simulink library "Simple_lib"  (R2018b)
settings: Solver=ode45  StartTime=0.0  StopTime=10.0  RelTol=1e-3  EnableMultiTasking=on
undefined symbols (not defined in the file or in its folder): Acceptance, beta, C, C_J, C_P, c_wall, dGain, DiscIntNeverNeededParam, Duplex, Electrical_lib, grab, h_fe, i, i3, K_T, Kman, KmanCE, mu_s, n_rev, R_arm, Simplex, systemTs, tau_0, TinIC, Ts, w_0, wallMass, Watch_lib
libraries: $bdroot x407, PlantUtilityBlockset_lib x30, peGeneralControl x22, simulink x11
(part 5 of 14)

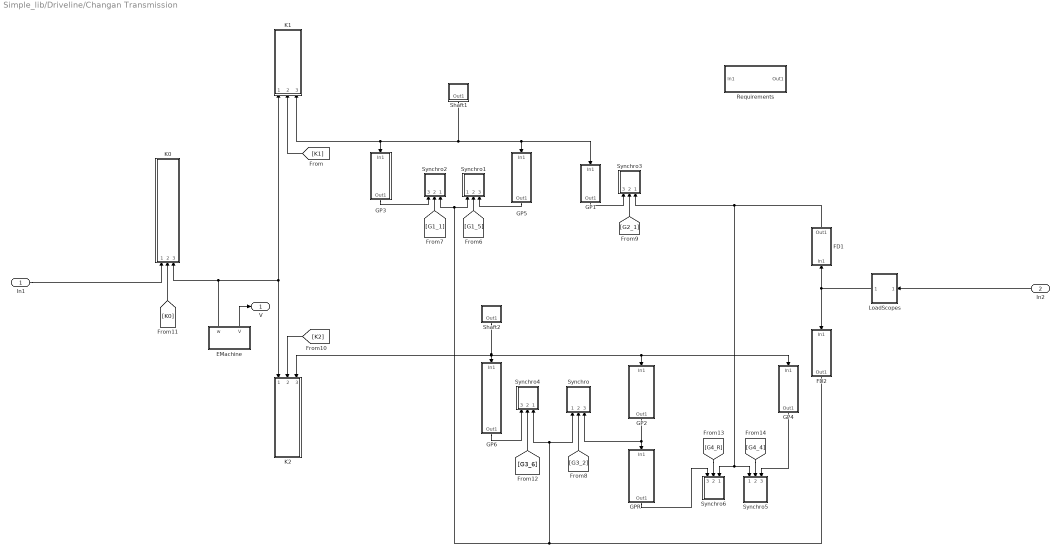
== system Simple_lib/Driveline/Changan Transmission ==
  In1 : Inport
  In2 : Inport  Port=2
  EMachine : Subsystem  AncestorBlock=PlantUtilityBlockset_lib/Electrical/EMachine
  FD1 : Subsystem  AncestorBlock=PlantUtilityBlockset_lib/Driveline/GearPair  mask{n_i=75, n_o=16}
      mask prompts: n_i "Number of input teeth"; n_o "Number of output teeth"
      mask Display:
      | plot([-n_i -5],[0 0]);
      | plot([5 n_o],[0 0]);
      | 
      | patch(-[3 3 5 5],[-1  1 1 -1]*(n_i+n_o));
      | patch([3 3 5 5],[-1  1 1 -1]*(n_i+n_o));
  FD2 : Subsystem  AncestorBlock=PlantUtilityBlockset_lib/Driveline/GearPair  mask{n_i=75, n_o=22}
      mask prompts: n_i "Number of input teeth"; n_o "Number of output teeth"
      mask Display:
      | plot([-n_i -5],[0 0]);
      | plot([5 n_o],[0 0]);
      | 
      | patch(-[3 3 5 5],[-1  1 1 -1]*(n_i+n_o));
      | patch([3 3 5 5],[-1  1 1 -1]*(n_i+n_o));
  GP1 : Subsystem  AncestorBlock=PlantUtilityBlockset_lib/Driveline/GearPair  mask{n_i=17, n_o=59}
      mask prompts: n_i "Number of input teeth"; n_o "Number of output teeth"
      mask Display:
      | plot([-n_i -5],[0 0]);
      | plot([5 n_o],[0 0]);
      | 
      | patch(-[3 3 5 5],[-1  1 1 -1]*(n_i+n_o));
      | patch([3 3 5 5],[-1  1 1 -1]*(n_i+n_o));
  GP2 : Subsystem  AncestorBlock=PlantUtilityBlockset_lib/Driveline/GearPair  mask{n_i=19, n_o=55}
      mask prompts: n_i "Number of input teeth"; n_o "Number of output teeth"
      mask Display:
      | plot([-n_i -5],[0 0]);
      | plot([5 n_o],[0 0]);
      | 
      | patch(-[3 3 5 5],[-1  1 1 -1]*(n_i+n_o));
      | patch([3 3 5 5],[-1  1 1 -1]*(n_i+n_o));
  GP3 : Subsystem  AncestorBlock=PlantUtilityBlockset_lib/Driveline/GearPair  mask{n_i=i3, n_o=49}
      mask prompts: n_i "Number of input teeth"; n_o "Number of output teeth"
      settings: AttributesFormatString=|
      | n_i = %<n_i>
      | n_o = %<n_o>
      mask Display:
      | plot([-n_i -5],[0 0]);
      | plot([5 n_o],[0 0]);
      | 
      | patch(-[3 3 5 5],[-1  1 1 -1]*(n_i+n_o));
      | patch([3 3 5 5],[-1  1 1 -1]*(n_i+n_o));
  "GP4 " : Subsystem  AncestorBlock=PlantUtilityBlockset_lib/Driveline/GearPair  mask{n_i=38, n_o=39}
      mask prompts: n_i "Number of input teeth"; n_o "Number of output teeth"
      mask Display:
      | plot([-n_i -5],[0 0]);
      | plot([5 n_o],[0 0]);
      | 
      | patch(-[3 3 5 5],[-1  1 1 -1]*(n_i+n_o));
      | patch([3 3 5 5],[-1  1 1 -1]*(n_i+n_o));
  GP5 : Subsystem  AncestorBlock=PlantUtilityBlockset_lib/Driveline/GearPair  mask{n_i=38, n_o=43}
      mask prompts: n_i "Number of input teeth"; n_o "Number of output teeth"
      mask Display:
      | plot([-n_i -5],[0 0]);
      | plot([5 n_o],[0 0]);
      | 
      | patch(-[3 3 5 5],[-1  1 1 -1]*(n_i+n_o));
      | patch([3 3 5 5],[-1  1 1 -1]*(n_i+n_o));
  GP6 : Subsystem  AncestorBlock=PlantUtilityBlockset_lib/Driveline/GearPair  mask{n_i=38, n_o=37}
      mask prompts: n_i "Number of input teeth"; n_o "Number of output teeth"
      mask Display:
      | plot([-n_i -5],[0 0]);
      | plot([5 n_o],[0 0]);
      | 
      | patch(-[3 3 5 5],[-1  1 1 -1]*(n_i+n_o));
      | patch([3 3 5 5],[-1  1 1 -1]*(n_i+n_o));
  GPR : Subsystem  AncestorBlock=PlantUtilityBlockset_lib/Driveline/GearPair  mask{n_i=55, n_o=48}
      mask prompts: n_i "Number of input teeth"; n_o "Number of output teeth"
      mask Display:
      | plot([-n_i -5],[0 0]);
      | plot([5 n_o],[0 0]);
      | 
      | patch(-[3 3 5 5],[-1  1 1 -1]*(n_i+n_o));
      | patch([3 3 5 5],[-1  1 1 -1]*(n_i+n_o));
  K0 : Subsystem  AncestorBlock="PlantUtilityBlockset_lib/Driveline/Pseudo Locking  Clutch"
      mask Display:
      | patch([0 1 1 0],[1 1 .9 .9]);
      | patch([0 1 1 0],-[1 1 .9 .9]);
  K1 : Subsystem  AncestorBlock="PlantUtilityBlockset_lib/Driveline/Pseudo Locking  Clutch"
      mask Display:
      | patch([0 1 1 0],[1 1 .9 .9]);
      | patch([0 1 1 0],-[1 1 .9 .9]);
  K2 : Subsystem  AncestorBlock="PlantUtilityBlockset_lib/Driveline/Pseudo Locking  Clutch"
      mask Display:
      | patch([0 1 1 0],[1 1 .9 .9]);
      | patch([0 1 1 0],-[1 1 .9 .9]);
  LoadScopes : Subsystem  AncestorBlock=PlantUtilityBlockset_lib/Utility/Scopes
      mask Display:
      | plot( [-1 1 1 -1 -1], [-1 -1 1 1 -1] );
      | plot( 0.6*[-1 1 1 -1 -1], 0.3 + 0.5*[-1 -1 1 1 -1] );
  Requirements : Subsystem
  Shaft1 : Subsystem  AncestorBlock=PlantUtilityBlockset_lib/Driveline/InertialState
      mask Display:
      | %color('white');
      | %plot([-1 4],[1 1]);
      | %plot([-1 4],[-1 -1]);
      | %color('black')
      | %plot([1 4],[0 0]);
      | plot([-1 -.9 -.5 0 .5 .9 1  .9  .5  0 -.5 -.9 -1],      [ 0  .5 .9 1 .9 .5 0 -.5 -.9 -1 -.9 -.5  0]);
      | %plot([4 4.5 4.5 4],[0 -0.25 0.25 0])
  Shaft2 : Subsystem  AncestorBlock=PlantUtilityBlockset_lib/Driveline/InertialState
      mask Display:
      | %color('white');
      | %plot([-1 4],[1 1]);
      | %plot([-1 4],[-1 -1]);
      | %color('black')
      | %plot([1 4],[0 0]);
      | plot([-1 -.9 -.5 0 .5 .9 1  .9  .5  0 -.5 -.9 -1],      [ 0  .5 .9 1 .9 .5 0 -.5 -.9 -1 -.9 -.5  0]);
      | %plot([4 4.5 4.5 4],[0 -0.25 0.25 0])
  Synchro : Subsystem
      mask Display:
      | %color('black')
      | %patch([-1 0 0 -1], [1 .9 1 .9]);
      | patch([1 1 0.4 -0.4 -1 -1], [1 .6 -.2 -.2 .6 1]);
      | patch([1 1 0.4 -0.4 -1 -1], -[1 0 .8 .8 0 1]);
      | color('white');
      | plot([-1 -1],[-1 1]);
      | plot([1 1],[-1 1]);
  Synchro1 : Subsystem
      mask Display:
      | %color('black')
      | %patch([-1 0 0 -1], [1 .9 1 .9]);
      | patch([1 1 0.4 -0.4 -1 -1], [1 .6 -.2 -.2 .6 1]);
      | patch([1 1 0.4 -0.4 -1 -1], -[1 0 .8 .8 0 1]);
      | color('white');
      | plot([-1 -1],[-1 1]);
      | plot([1 1],[-1 1]);
  Synchro2 : Subsystem
      mask Display:
      | %color('black')
      | %patch([-1 0 0 -1], [1 .9 1 .9]);
      | patch([1 1 0.4 -0.4 -1 -1], [1 .6 -.2 -.2 .6 1]);
      | patch([1 1 0.4 -0.4 -1 -1], -[1 0 .8 .8 0 1]);
      | color('white');
      | plot([-1 -1],[-1 1]);
      | plot([1 1],[-1 1]);
  Synchro3 : Subsystem
      mask Display:
      | %color('black')
      | %patch([-1 0 0 -1], [1 .9 1 .9]);
      | patch([1 1 0.4 -0.4 -1 -1], [1 .6 -.2 -.2 .6 1]);
      | patch([1 1 0.4 -0.4 -1 -1], -[1 0 .8 .8 0 1]);
      | color('white');
      | plot([-1 -1],[-1 1]);
      | plot([1 1],[-1 1]);
  Synchro4 : Subsystem
      mask Display:
      | %color('black')
      | %patch([-1 0 0 -1], [1 .9 1 .9]);
      | patch([1 1 0.4 -0.4 -1 -1], [1 .6 -.2 -.2 .6 1]);
      | patch([1 1 0.4 -0.4 -1 -1], -[1 0 .8 .8 0 1]);
      | color('white');
      | plot([-1 -1],[-1 1]);
      | plot([1 1],[-1 1]);
  Synchro5 : Subsystem
      mask Display:
      | %color('black')
      | %patch([-1 0 0 -1], [1 .9 1 .9]);
      | patch([1 1 0.4 -0.4 -1 -1], [1 .6 -.2 -.2 .6 1]);
      | patch([1 1 0.4 -0.4 -1 -1], -[1 0 .8 .8 0 1]);
      | color('white');
      | plot([-1 -1],[-1 1]);
      | plot([1 1],[-1 1]);
  Synchro6 : Subsystem
      mask Display:
      | %color('black')
      | %patch([-1 0 0 -1], [1 .9 1 .9]);
      | patch([1 1 0.4 -0.4 -1 -1], [1 .6 -.2 -.2 .6 1]);
      | patch([1 1 0.4 -0.4 -1 -1], -[1 0 .8 .8 0 1]);
      | color('white');
      | plot([-1 -1],[-1 1]);
      | plot([1 1],[-1 1]);
  V : Outport
  wires:
  EMachine/2(w) -> K2/1(w_in), K1/1(w_in), K0/3(w_out)
  Shaft1/1(Out1) -> K1/3(w_out), GP3/1(In1), GP1/1(In1), GP5/1(In1)
  GP3/1(Out1) -> Synchro2/3(w_out)
  GP1/1(Out1) -> Synchro3/3(w_out)
  GP2/1(Out1) -> GPR/1(In1), Synchro/3(w_out)
  [K1] -> K1/2(cap)
  [K0] -> K0/2(cap)
  [K2] -> K2/2(cap)
  [G2_1] -> Synchro3/2(cap)
  [G3_2] -> Synchro/2(cap)
  [G1_1] -> Synchro2/2(cap)
  [G1_5] -> Synchro1/2(cap)
  GP5/1(Out1) -> Synchro1/3(w_out)
  FD1/1(Out1) -> Synchro6/1(w_in), Synchro5/1(w_in), Synchro3/1(w_in)
  GP6/1(Out1) -> Synchro4/3(w_out)
  [G3_6] -> Synchro4/2(cap)
  Shaft2/1(Out1) -> K2/3(w_out), "GP4 "/1(In1), GP2/1(In1), GP6/1(In1)
  "GP4 "/1(Out1) -> Synchro5/3(w_out)
  [G4_4] -> Synchro5/2(cap)
  [G4_R] -> Synchro6/2(cap)
  GPR/1(Out1) -> Synchro6/3(w_out)
  EMachine/1(V) -> V/1
  FD2/1(Out1) -> Synchro1/1(w_in), Synchro2/1(w_in), Synchro4/1(w_in), Synchro/1(w_in)
  LoadScopes/1(Out1) -> FD1/1(In1), FD2/1(In1)
  In2/1 -> LoadScopes/1(In1)
  In1/1 -> K0/1(w_in)

== system Simple_lib/Driveline/Clutch ==
  note: {\bfSimple Clutch}
      | Clutch torque is a sigmoidal function of speed difference.
  K : Inport
  in : Inport  Port=2
  T : Inport  Port=3
  Friction : $bdroot/Rotational/Friction  grab=.03  s=.2  Ki=1
  Saturation : Saturate  UpperLimit=inf  LowerLimit=0
      settings: AttributesFormatString=|
      | %<UpperLimit>
      | %<LowerLimit>
  Terminator : Terminator
  from : $bdroot/Rotational/Lump  w_0=w_0  max_accel=inf  conserved_quantity_name=Momentum  energy_name=Energy
  out : Outport
  wires:
  K/1 -> Saturation/1
  in/1 -> Friction/1
  T/1 -> Terminator/1
  Saturation/1 -> Friction/2
  from/1 -> out/1, Friction/3

== system Simple_lib/Driveline/Compliant Wheel_wv ==
  w : Inport
  r : Inport  Port=2
  Bus Creator : BusCreator  Inputs=2
  Bus Selector : BusSelector  OutputSignals=F,M
  Times : Product  Inputs=**
  Times1 : Product  Inputs=**
  Times2 : Product  Inputs=**
  _out : $bdroot/Translational/_out  Tag=Electrical  Level=v  Flow=F
  in : $bdroot/Rotational/_in  Level=w  Flow=Tq
  v : Outport
  wires:
  Bus Selector/1 -> Times1/2  "<F>"
  Bus Selector/2 -> Times2/2  "<M>"
  in/1 -> Times/1
  Times/1 -> _out/1
  _out/2 -> Bus Selector/1
  Bus Creator/1 -> in/2
  w/1 -> in/1
  _out/1 -> v/1
  r/1 -> Times/2, Times1/1, Times2/1
  Times1/1 -> Bus Creator/1  "tau"
  Times2/1 -> Bus Creator/2  "J"

== system Simple_lib/Driveline/Differential ==
  In1 : Inport
  BiGain : $bdroot/Rotational/BiGain  k_level=-1  k_flow=-1
      settings: AttributesFormatString="%<k_flow>   %<k_pot>"
  First : $bdroot/Driveline/GearPair  n_i=r*100  n_o=100
  InertialState : $bdroot/Rotational/Lump  w_0=0  max_accel=inf
  Sum : Sum  Inputs=|++
  Sum1 : Sum  Inputs=|++
  Out1 : Outport
  Out2 : Outport  Port=2
  wires:
  BiGain/1 -> Sum/2
  Sum1/1 -> Out2/1
  Sum/1 -> Out1/1
  InertialState/1 -> BiGain/1, Sum1/2
  First/1 -> Sum1/1, Sum/1
  In1/1 -> First/1

== system Simple_lib/Driveline/Drag ==
  In1 : Inport
  A : Gain  Gain=2
  Bus Creator : BusCreator  Inputs=2
  Bus Selector : BusSelector  OutputSignals=i
  Cd : Gain  Gain=0.3
  Gain2 : Gain  Gain=-1/2
  Ground : Ground
  Multiply : Product  Inputs=3
  Sign : Signum
  _at : $bdroot/Translational/_in  Level=v  Flow=F
  rho : Gain
  wires:
  In1/1 -> Bus Selector/1
  _at/1 -> Multiply/2, Multiply/3, Sign/1
  Sign/1 -> Multiply/1
  Multiply/1 -> Gain2/1
  Cd/1 -> A/1
  A/1 -> rho/1
  Gain2/1 -> Cd/1
  rho/1 -> Bus Creator/1  "F"
  Bus Selector/1 -> _at/1  "<i>"
  Bus Creator/1 -> _at/2
  Ground/1 -> Bus Creator/2  "M"

== system Simple_lib/Driveline/EndStop ==
  In1 : Inport
  In2 : Inport  Port=2
  1/R1 : Gain  Gain=-1
  1/R2 : Gain  Gain=-1
  1/R3 : Gain  Gain=k
  1/R4 : Gain  Gain=k
  Compare To Zero : simulink/Logic and Bit Operations/Compare To Zero  relop=~=  OutDataTypeStr=boolean
  Dead Zone : DeadZone  LowerValue=-0.01  UpperValue=0.31  SaturateOnIntegerOverflow=on
  Discrete-Time Integrator1 : DiscreteIntegrator  gainval=1  SampleTime=Ts  ICPrevOutput=DiscIntNeverNeededParam  ICPrevScaledInput=DiscIntNeverNeededParam
  Input : $bdroot/Utility/Input  Level=V  Flow=I
  Input1 : $bdroot/Utility/Input  Level=V  Flow=I
  Multiply : Product
  Sum : Sum  Inputs=+|+
  Sum1 : Sum  Inputs=|++
  wires:
  Compare To Zero/1 -> Multiply/1
  Multiply/1 -> 1/R4/1
  1/R4/1 -> Sum1/2
  1/R3/1 -> Sum1/1
  1/R1/1 -> Input1/2
  Input1/1 -> Sum/2
  In2/1 -> Input1/1
  Sum/1 -> Discrete-Time Integrator1/1, Multiply/2
  1/R2/1 -> Sum/1
  Input/1 -> 1/R2/1
  In1/1 -> Input/1
  Discrete-Time Integrator1/1 -> Dead Zone/1
  Dead Zone/1 -> 1/R3/1, Compare To Zero/1
  Sum1/1 -> 1/R1/1, Input/2

== system Simple_lib/Driveline/Engine ==
  Ped : Inport
  Crank : $bdroot/Driveline/MeanTorqueMapModel  SystemSampleTime=-1
  Flywheel : $bdroot/Rotational/Lump  w_0=w_0  max_accel=inf  conserved_quantity_name=Momentum  energy_name=Energy
  Inertia : $bdroot/Rotational/Inertia  I=0.1
      settings: AttributesFormatString=%<I> kgm^2
  M : $bdroot/Rotational/M1  SystemSampleTime=-1
  w : Outport
  wires:
  Flywheel/1 -> Inertia/1, M/1, Crank/2
  M/1 -> w/1
  Ped/1 -> Crank/1

== system Simple_lib/Driveline/FailingClutch ==
  note: {\bfClutch}
      | Passes the smaller of the input torque and its (non-negative) capacity K (Kappa).
  K : Inport
  in : Inport  Port=2
  T : Inport  Port=3
  Abs1 : Abs
  Complex to Real-Imag1 : ComplexToRealImag
  Discrete-Time Integrator : DiscreteIntegrator  gainval=1  InitialCondition=w_0  SampleTime=-1  LowerSaturationLimit=0  ICPrevOutput=DiscIntNeverNeededParam  ICPrevScaledInput=DiscIntNeverNeededParam
  Filtered Derivative (Discrete or Continuous) : peGeneralControl/Filtered Derivative (Discrete or Continuous)  K=1  T=Ts*20  B=inf  A=-inf  minRatio=10  Ts=-1
  Gain : Gain  Gain=-1
  Gain1 : Gain  Gain=+1
  Ground : Ground
  MinMax1 : MinMax  Inputs=2
  Multiply : Product  Inputs=*/
  Product1 : Product
  Product2 : Product
  Real-Imag to Complex1 : RealImagToComplex
  Saturation1 : Saturate  UpperLimit=inf  LowerLimit=0
      settings: AttributesFormatString=|
      | %<UpperLimit>
      | %<LowerLimit>
  Sign1 : Signum
  Sum1 : Sum  Inputs=|-+
  Terminator : Terminator
  _in : $bdroot/Utility/Input  Level=w  Flow=Tq
  _out : $bdroot/Utility/Output  Tag=Electrical  Level=w  Flow=Tq
  out : Outport
  wires:
  Gain/1 -> Discrete-Time Integrator/1  "dw_on"
  Filtered Derivative (Discrete or Continuous)/1 -> Gain1/1
  Product2/1 -> Sum1/1  "Tq_I"
  Gain1/1 -> Product2/1  "dw_in"
  Complex to Real-Imag1/2 -> Product2/2, Multiply/2  "Inertia"
  Multiply/1 -> Gain/1
  Ground/1 -> Real-Imag to Complex1/2
  Sum1/1 -> Sign1/1, Abs1/1  "Tq_needed"
  Saturation1/1 -> MinMax1/1
  Sign1/1 -> Product1/2
  Abs1/1 -> MinMax1/2
  K/1 -> Saturation1/1
  MinMax1/1 -> Product1/1
  _out/2 -> Complex to Real-Imag1/1
  Real-Imag to Complex1/1 -> _in/2
  _out/1 -> out/1
  _in/1 -> Filtered Derivative (Discrete or Continuous)/1  "w_in"
  Discrete-Time Integrator/1 -> _out/1  "w_out"
  Product1/1 -> Multiply/1, Real-Imag to Complex1/1  "Tq_trn"
  in/1 -> _in/1
  T/1 -> Terminator/1
  Complex to Real-Imag1/1 -> Sum1/2  "Tq_Re"

== system Simple_lib/Driveline/GearPair ==
  In1 : Inport
  Bus Creator : BusCreator  Inputs=2
  Bus Selector : BusSelector  OutputSignals=tau,J
  _in : $bdroot/Rotational/_in  Level=w  Flow=tau
  _out : $bdroot/Rotational/_out  Tag=Electrical  Level=w  Flow=tau
  ratio : Gain  Gain=n_i/n_o
  ratio1 : Gain  Gain=n_i/n_o
  ratio2 : Gain  Gain=n_i/n_o
  speed ratio : Gain  Gain=n_i/n_o
  Out1 : Outport
  wires:
  _in/1 -> speed ratio/1
  speed ratio/1 -> _out/1
  Bus Creator/1 -> _in/2
  In1/1 -> _in/1
  _out/1 -> Out1/1
  _out/2 -> Bus Selector/1
  Bus Selector/1 -> ratio/1  "<tau>"
  ratio/1 -> Bus Creator/1  "tau"
  Bus Selector/2 -> ratio2/1  "<J>"
  ratio2/1 -> ratio1/1
  ratio1/1 -> Bus Creator/2  "J"

== system Simple_lib/Driveline/GearPair  ==
  In1 : Inport
  Pull : PlantUtilityBlockset_lib/Utility/Pull  Tag=Electrical  SystemSampleTime=-1
  Push : PlantUtilityBlockset_lib/Utility/Push  SystemSampleTime=-1
  ratio : Gain  Gain=n_i/n_o
  speed ratio : Gain  Gain=n_i/n_o
  Out1 : Outport
  wires:
  Pull/1 -> Out1/1
  In1/1 -> Push/1
  ratio/1 -> Push/2
  Pull/2 -> ratio/1
  speed ratio/1 -> Pull/1
  Push/1 -> speed ratio/1

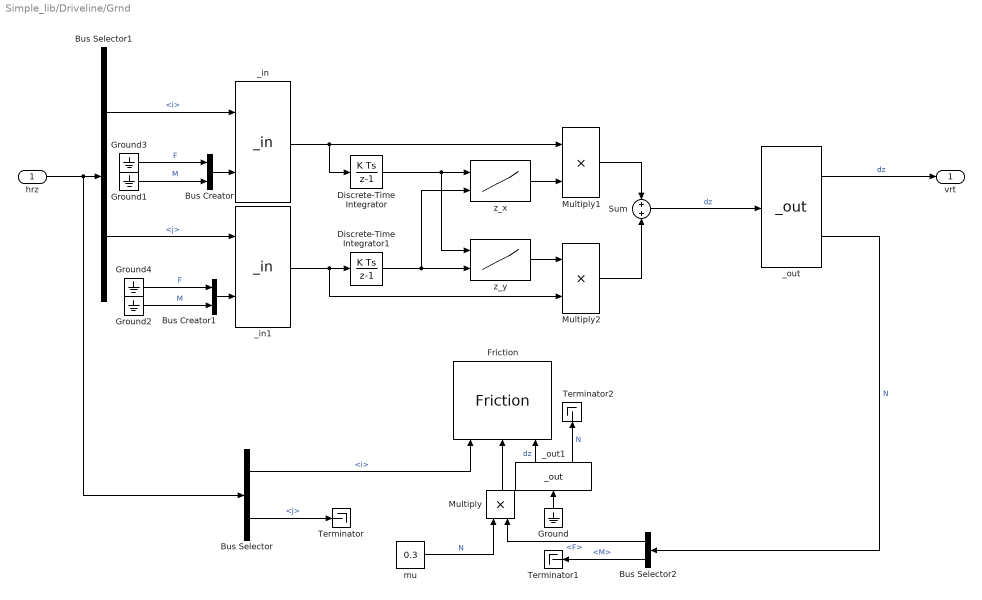
== system Simple_lib/Driveline/Grnd ==
  hrz : Inport
  Bus Creator : BusCreator  Inputs=2
  Bus Creator1 : BusCreator  Inputs=2
  Bus Selector : BusSelector  OutputSignals=i,j
  Bus Selector1 : BusSelector  OutputSignals=i,j
  Bus Selector2 : BusSelector  OutputSignals=F,M
  Discrete-Time Integrator : DiscreteIntegrator  SampleTime=-1  ICPrevOutput=DiscIntNeverNeededParam  ICPrevScaledInput=DiscIntNeverNeededParam
  Discrete-Time Integrator1 : DiscreteIntegrator  SampleTime=-1  ICPrevOutput=DiscIntNeverNeededParam  ICPrevScaledInput=DiscIntNeverNeededParam
  Friction : $bdroot/Translational/Friction  grab=0.1  s=1  Ki=0
  Ground{,1..4} (5 alike) : Ground
  Multiply : Product
  Multiply1 : Product
  Multiply2 : Product
  Sum : Sum  Inputs=+|+
  Terminator : Terminator
  Terminator1 : Terminator
  Terminator2 : Terminator
  _in : $bdroot/Translational/_in  Level=v  Flow=F
  _in1 : $bdroot/Translational/_in  Level=v  Flow=F
  _out : $bdroot/Translational/_out  Tag=Electrical  Level=v  Flow=F
  _out1 : $bdroot/Translational/_out  Tag=Electrical  Level=v  Flow=F
  mu : Constant  Value=0.3
  z_x : Lookup_n-D  BreakpointsForDimension1=[1:3]  BreakpointsForDimension2=[1:3]  Table=[4 5 6;16 19 20;10 18 23]*0  InternalRulePriority=Speed  RndMeth=Simplest  InputSameDT=on
  z_y : Lookup_n-D  BreakpointsForDimension1=[1:3]  BreakpointsForDimension2=[1:3]  Table=[4 5 6;16 19 20;10 18 23]*0  InternalRulePriority=Speed  RndMeth=Simplest  InputSameDT=on
  vrt : Outport
  wires:
  Sum/1 -> _out/1  "dz"
  Multiply2/1 -> Sum/2
  Multiply1/1 -> Sum/1
  z_y/1 -> Multiply2/1
  z_x/1 -> Multiply1/2
  Discrete-Time Integrator1/1 -> z_y/2, z_x/2
  Discrete-Time Integrator/1 -> z_x/1, z_y/1
  _in1/1 -> Multiply2/2, Discrete-Time Integrator1/1
  _in/1 -> Discrete-Time Integrator/1, Multiply1/1
  Ground1/1 -> Bus Creator/2  "M"
  Ground/1 -> _out1/1
  Bus Selector/1 -> Friction/1  "<i>"
  hrz/1 -> Bus Selector/1, Bus Selector1/1
  mu/1 -> Multiply/1  "N"
  _out/1 -> vrt/1  "dz"
  _out/2 -> Bus Selector2/1  "N"
  Multiply/1 -> Friction/2
  Bus Selector/2 -> Terminator/1  "<j>"
  Bus Selector2/1 -> Multiply/2  "<F>"
  Bus Selector2/2 -> Terminator1/1  "<M>"
  Bus Selector1/1 -> _in/1  "<i>"
  Bus Selector1/2 -> _in1/1  "<j>"
  _out1/1 -> Friction/3  "dz"
  _out1/2 -> Terminator2/1  "N"
  Bus Creator/1 -> _in/2
  Ground3/1 -> Bus Creator/1  "F"
  Bus Creator1/1 -> _in1/2
  Ground4/1 -> Bus Creator1/1  "F"
  Ground2/1 -> Bus Creator1/2  "M"

== system Simple_lib/Driveline/Hub ==
  in : Inport
  Brake : $bdroot/Driveline/Brake  SystemSampleTime=-1
  Bus Creator : BusCreator  Inputs=2
  Bus Creator1 : BusCreator  Inputs=3
  Bus Selector : BusSelector  OutputSignals=str,brk,rtn,trn
  Bus Selector1 : BusSelector  OutputSignals=i,j,k
  Ground : Ground
  I : $bdroot/Rotational/Inertia  I=1
  Inertia : $bdroot/Translational/Sink  m=0.01
  Terminator2 : Terminator
  out : Outport
  wires:
  Bus Creator1/1 -> Bus Creator/2  "trn"
  Bus Selector1/3 -> Inertia/1, Bus Creator1/3  "<k>"
  Bus Selector1/2 -> Bus Creator1/2  "<j>"
  Bus Selector1/1 -> Bus Creator1/1  "<i>"
  Bus Selector/4 -> Bus Selector1/1  "<trn>"
  Bus Creator/1 -> out/1  "hub"
  in/1 -> Bus Selector/1
  Bus Selector/2 -> Brake/1  "<brk>"
  Ground/1 -> Brake/3
  Bus Selector/3 -> Brake/2, I/1, Bus Creator/1  "<rtn>"
  Bus Selector/1 -> Terminator2/1  "<str>"

== system Simple_lib/Driveline/Inverter_F ==
  note: NB currently 100% efficient!
  Vdc : Inport
  P_req : Inport  Port=2
  Vac : Inport  Port=3
  DivideSafely_1 : Subsystem
  DivideSafely_2 : Subsystem
  Preq_F : Scope
  Simplex : Subsystem  Tag=Electrical  AncestorBlock=PlantUtilityBlockset_lib/Utility/Push  InitFcn=initSimplex
      mask Display:
      | color('white')
      | plot([0 3], [2 2])
      | plot([0 3], [-2 -2])
      | color('black')
      | 
      | plot([0 2 2 3], [1 1 0 0])
      | plot([1 3 2 1 0 2], [0.6 0.6 0.4 0.6 0.4 0.4])
      | patch([1 3 2],[0.6 0.6 0.4],[0,0,0])
      | plot([0 1 1], [1 1 0.6])
      | plot([1 1 0], [0.4 -1 -1])
  Simplex1 : Subsystem  Tag=Electrical  AncestorBlock=PlantUtilityBlockset_lib/Utility/Push  InitFcn=initSimplex
      mask Display:
      | color('white')
      | plot([0 3], [2 2])
      | plot([0 3], [-2 -2])
      | color('black')
      | 
      | plot([0 2 2 3], [1 1 0 0])
      | plot([1 3 2 1 0 2], [0.6 0.6 0.4 0.6 0.4 0.4])
      | patch([1 3 2],[0.6 0.6 0.4],[0,0,0])
      | plot([0 1 1], [1 1 0.6])
      | plot([1 1 0], [0.4 -1 -1])
  wires:
  Vac/1 -> Simplex/1(InPot)
  Vdc/1 -> Simplex1/1(InPot)
  Simplex1/1(OutPot) -> DivideSafely_1/1(den)
  Simplex/1(OutPot) -> DivideSafely_2/2(den)
  DivideSafely_1/1(rat) -> Simplex1/2(InFlow)
  DivideSafely_2/1(rat) -> Simplex/2(InFlow)
  P_req/1 -> Preq_F/1, DivideSafely_1/2(num), DivideSafely_2/1(num)

== system Simple_lib/Driveline/Inverter_R ==
  note: NB currently 100% efficient!
  note: NB currently 100% efficient!
  Vdc : Inport
  P_req : Inport  Port=2
  Vac : Inport  Port=3
  DivideSafely_1 : Subsystem
  DivideSafely_2 : Subsystem
  Preq_R : Scope
  Simplex : Subsystem  Tag=Electrical  AncestorBlock=PlantUtilityBlockset_lib/Utility/Push  InitFcn=initSimplex
      mask Display:
      | color('white')
      | plot([0 3], [2 2])
      | plot([0 3], [-2 -2])
      | color('black')
      | 
      | plot([0 2 2 3], [1 1 0 0])
      | plot([1 3 2 1 0 2], [0.6 0.6 0.4 0.6 0.4 0.4])
      | patch([1 3 2],[0.6 0.6 0.4],[0,0,0])
      | plot([0 1 1], [1 1 0.6])
      | plot([1 1 0], [0.4 -1 -1])
  Simplex1 : Subsystem  Tag=Electrical  AncestorBlock=PlantUtilityBlockset_lib/Utility/Push  InitFcn=initSimplex
      mask Display:
      | color('white')
      | plot([0 3], [2 2])
      | plot([0 3], [-2 -2])
      | color('black')
      | 
      | plot([0 2 2 3], [1 1 0 0])
      | plot([1 3 2 1 0 2], [0.6 0.6 0.4 0.6 0.4 0.4])
      | patch([1 3 2],[0.6 0.6 0.4],[0,0,0])
      | plot([0 1 1], [1 1 0.6])
      | plot([1 1 0], [0.4 -1 -1])
  Test : Scope
  wires:
  Vac/1 -> Simplex/1(InPot)
  Vdc/1 -> Simplex1/1(InPot)
  Simplex1/1(OutPot) -> DivideSafely_1/1(den)
  Simplex/1(OutPot) -> DivideSafely_2/2(den)
  DivideSafely_1/1(rat) -> Test/1, Simplex1/2(InFlow)
  DivideSafely_2/1(rat) -> Simplex/2(InFlow)
  P_req/1 -> Preq_R/1, DivideSafely_1/2(num), DivideSafely_2/1(num)

== system Simple_lib/Driveline/KellyClutch ==
  note: {\bfSeries Clutch}
      | Passes the smaller of the input torque and its capacity.
  K : Inport
  w_in : Inport  Port=2
  T : Inport  Port=3
  Abs : Abs
  Bus Selector : BusSelector  OutputSignals=tau,J
  Discrete-Time Integrator : DiscreteIntegrator  gainval=k_clutch  InitialCondition=max(w_drop,0)  SampleTime=Ts  LimitOutput=on  LowerSaturationLimit=0  ICPrevOutput=DiscIntNeverNeededParam  ICPrevScaledInput=DiscIntNeverNeededParam
  Divide : Product  Inputs=*/
  MinMax : MinMax  Inputs=2
  Product : Product
  Real-Imag to Complex : RealImagToComplex
  Saturation : Saturate  UpperLimit=inf  LowerLimit=0
      settings: AttributesFormatString=|
      | %<UpperLimit>
      | %<LowerLimit>
  Sign : Signum
  Sum : Sum  Inputs=|+-
  Sum1 : Sum  Inputs=|-+
  Terminator : Terminator
  _in : $bdroot/Rotational/_in  Level=w  Flow=tau
  _out : $bdroot/Rotational/_out  Tag=Electrical  Level=w  Flow=tau
  w_out : Outport
  wires:
  ? -> Real-Imag to Complex/2
  Real-Imag to Complex/1 -> _in/2
  _out/1 -> w_out/1
  _in/1 -> Sum/1
  Sum/1 -> _out/1
  MinMax/1 -> Product/2
  K/1 -> Saturation/1
  Abs/1 -> MinMax/1
  Product/1 -> Real-Imag to Complex/1
  Sign/1 -> Product/1
  Sum1/1 -> Divide/1
  Discrete-Time Integrator/1 -> Sum/2
  w_in/1 -> _in/1
  Saturation/1 -> Sum1/1, MinMax/2
  T/1 -> Terminator/1
  _out/2 -> Bus Selector/1, Abs/1, Sign/1
  Bus Selector/1 -> Sum1/2  "<tau>"
  Divide/1 -> Discrete-Time Integrator/1
  Bus Selector/2 -> Divide/2  "<J>"

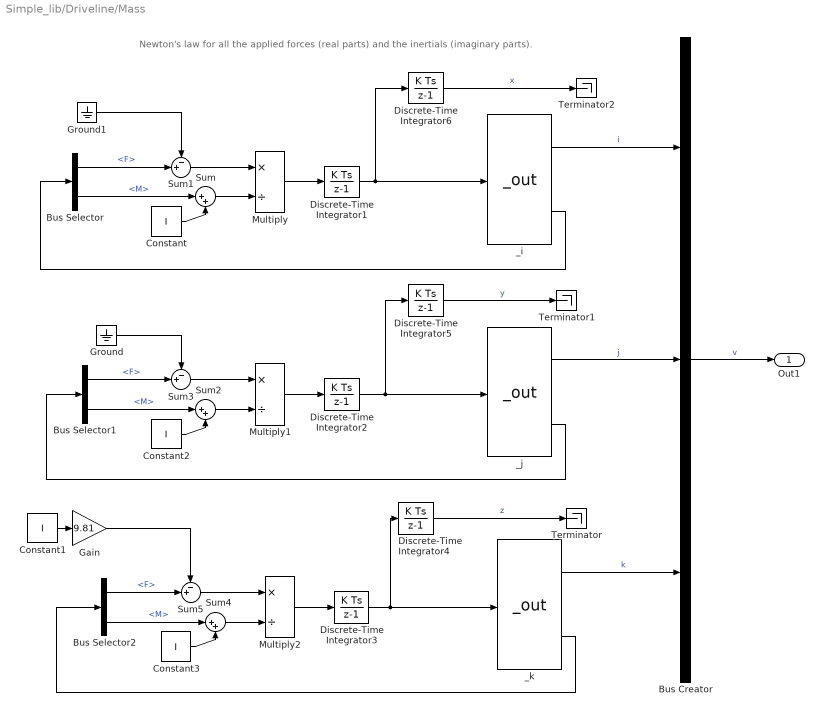
== system Simple_lib/Driveline/Mass ==
  note: Newton's law for all the applied forces (real parts) and the inertials (imaginary parts).
  Bus Creator : BusCreator  Inputs=3
  Bus Selector : BusSelector  OutputSignals=F,M
  Bus Selector1 : BusSelector  OutputSignals=F,M
  Bus Selector2 : BusSelector  OutputSignals=F,M
  Constant{,1..3} (4 alike) : Constant  Value=I
  Discrete-Time Integrator1 : DiscreteIntegrator  gainval=1  InitialCondition=v_0(1)  SampleTime=-1  ICPrevOutput=DiscIntNeverNeededParam  ICPrevScaledInput=DiscIntNeverNeededParam
  Discrete-Time Integrator2 : DiscreteIntegrator  gainval=1  InitialCondition=v_0(2)  SampleTime=-1  ICPrevOutput=DiscIntNeverNeededParam  ICPrevScaledInput=DiscIntNeverNeededParam
  Discrete-Time Integrator{3..6} (4 alike) : DiscreteIntegrator  gainval=1  InitialCondition=v_0(3)  SampleTime=-1  ICPrevOutput=DiscIntNeverNeededParam  ICPrevScaledInput=DiscIntNeverNeededParam
  Gain : Gain  Gain=9.81
  Ground : Ground
  Ground1 : Ground
  Multiply : Product  Inputs=*/
  Multiply1 : Product  Inputs=*/
  Multiply2 : Product  Inputs=*/
  Sum : Sum  Inputs=|++
  Sum1 : Sum  Inputs=-+|
  Sum2 : Sum  Inputs=|++
  Sum3 : Sum  Inputs=-+|
  Sum4 : Sum  Inputs=|++
  Sum5 : Sum  Inputs=-+|
  Terminator : Terminator
  Terminator1 : Terminator
  Terminator2 : Terminator
  _i : $bdroot/Translational/_out  Tag=Electrical  Level=v  Flow=F
  _j : $bdroot/Translational/_out  Tag=Electrical  Level=v  Flow=F
  _k : $bdroot/Translational/_out  Tag=Electrical  Level=v  Flow=F
  Out1 : Outport
  wires:
  Discrete-Time Integrator6/1 -> Terminator2/1  "x"
  Discrete-Time Integrator5/1 -> Terminator1/1  "y"
  Discrete-Time Integrator4/1 -> Terminator/1  "z"
  Ground1/1 -> Sum1/1
  Constant1/1 -> Gain/1
  Gain/1 -> Sum5/1
  Ground/1 -> Sum3/1
  Bus Selector2/2 -> Sum4/1  "<M>"
  Sum5/1 -> Multiply2/1
  Sum4/1 -> Multiply2/2
  Constant3/1 -> Sum4/2
  _k/2 -> Bus Selector2/1
  Bus Selector2/1 -> Sum5/2  "<F>"
  Discrete-Time Integrator3/1 -> _k/1, Discrete-Time Integrator4/1
  Multiply2/1 -> Discrete-Time Integrator3/1
  Bus Selector1/2 -> Sum2/1  "<M>"
  Sum3/1 -> Multiply1/1
  Sum2/1 -> Multiply1/2
  Constant2/1 -> Sum2/2
  _j/2 -> Bus Selector1/1
  Bus Selector1/1 -> Sum3/2  "<F>"
  Discrete-Time Integrator2/1 -> _j/1, Discrete-Time Integrator5/1
  Multiply1/1 -> Discrete-Time Integrator2/1
  _i/1 -> Bus Creator/1  "i"
  _j/1 -> Bus Creator/2  "j"
  Bus Creator/1 -> Out1/1  "v"
  _k/1 -> Bus Creator/3  "k"
  Multiply/1 -> Discrete-Time Integrator1/1
  Discrete-Time Integrator1/1 -> _i/1, Discrete-Time Integrator6/1
  Constant/1 -> Sum/2
  Bus Selector/1 -> Sum1/2  "<F>"
  _i/2 -> Bus Selector/1
  Sum/1 -> Multiply/2
  Sum1/1 -> Multiply/1
  Bus Selector/2 -> Sum/1  "<M>"

== system Simple_lib/Driveline/MeanTorqueMapModel ==
  Ped : Inport
  w : Inport  Port=2
  Bus Creator : BusCreator  Inputs=3
  Gain : Gain  Gain=-1
  Ground : Ground
  Ground1 : Ground
  MeanTorqueMap : Lookup2D  RowIndex=[0,20,30,40,50,60,70,80,90,100]  ColumnIndex=[800,1200,1600,2000,2400,2800,3200,3600,4000,4400,4800]  Table=reshape([-40,215,230,250,245,267,267,267,267,267,-44,117,208,260,279,290,297,301,301,301,-49,85,178,241,282,293,305,308,312,312,-53,66,148,219,275,297,305,312,319,319,-57,44,122,193,260,290,305,319,327,327,-62,29,104,167,238,275,301,323,327,334,-64,10,85,152,223,260,293,319,327,334,-70,-2,66,133,208,256,282,316,327,334,-75,-13,48,119,189,234,267,297,312,319,-79,-22,33,96,171,212,249,279,293,305,-82,-32,18,85,152,193,226,253,267,275],10,11)
  SItoRPM : Gain  Gain=2*pi/60
  _at : $bdroot/Rotational/_in  Level=w  Flow=Tq
  wires:
  Gain/1 -> Bus Creator/1  "tau"
  Ground1/1 -> Bus Creator/2  "c"
  _at/1 -> SItoRPM/1  "w"
  MeanTorqueMap/1 -> Gain/1  "tau_out"
  SItoRPM/1 -> MeanTorqueMap/2  "w_rpm"
  Ground/1 -> Bus Creator/3  "J"
  w/1 -> _at/1  "w"
  Bus Creator/1 -> _at/2
  Ped/1 -> MeanTorqueMap/1

== system Simple_lib/Driveline/Pseudo Locking Clutch ==
  w_in : Inport
  cap : Inport  Port=2
  w_out : Inport  Port=3
  1/R1 : Gain  Gain=-1
  1/R4 : Gain  Gain=-1
  Delay : Delay  DelayLength=1  InitialCondition=0
  Dw : Scope
  Dynamic Friction : Subsystem
  Push_in : Subsystem  AncestorBlock=PlantUtilityBlockset_lib/Utility/Push  InitFcn=initSimplex
      mask Display:
      | color('white')
      | plot([0 3], [2 2])
      | plot([0 3], [-2 -2])
      | color('black')
      | 
      | plot([0 2 2 3], [1 1 0 0])
      | plot([1 3 2 1 0 2], [0.6 0.6 0.4 0.6 0.4 0.4])
      | patch([1 3 2],[0.6 0.6 0.4],[0,0,0])
      | plot([0 1 1], [1 1 0.6])
      | plot([1 1 0], [0.4 -1 -1])
  Push_out : Subsystem  AncestorBlock=PlantUtilityBlockset_lib/Utility/Push  InitFcn=initSimplex
      mask Display:
      | color('white')
      | plot([0 3], [2 2])
      | plot([0 3], [-2 -2])
      | color('black')
      | 
      | plot([0 2 2 3], [1 1 0 0])
      | plot([1 3 2 1 0 2], [0.6 0.6 0.4 0.6 0.4 0.4])
      | patch([1 3 2],[0.6 0.6 0.4],[0,0,0])
      | plot([0 1 1], [1 1 0.6])
      | plot([1 1 0], [0.4 -1 -1])
  Static Friction : Subsystem
  Sum : Sum  Inputs=+|+
  Sum1 : Sum  Inputs=+|+
  Tq_Dyn : Scope
  Tq_stat : Scope
  Tq_trans : Scope
  capacity : Scope
  wires:
  1/R1/1 -> Push_out/2(InFlow)
  cap/1 -> Static Friction/1(cap), Dynamic Friction/2(cap), capacity/1
  Delay/1 -> Static Friction/4(Tq), Tq_trans/1
  Static Friction/1(Tq_stat) -> Sum1/2, Tq_stat/1
  Dynamic Friction/1(Tq_dyn) -> Sum1/1, Tq_Dyn/1
  Push_in/1(OutPot) -> 1/R4/1
  Push_out/1(OutPot) -> Sum/2, Static Friction/3(w)
  Sum/1 -> Static Friction/2(Dw), Dw/1, Dynamic Friction/1(Dw)
  Sum1/1 -> Push_in/2(InFlow), Delay/1, 1/R1/1
  1/R4/1 -> Sum/1
  w_in/1 -> Push_in/1(InPot)
  w_out/1 -> Push_out/1(InPot)

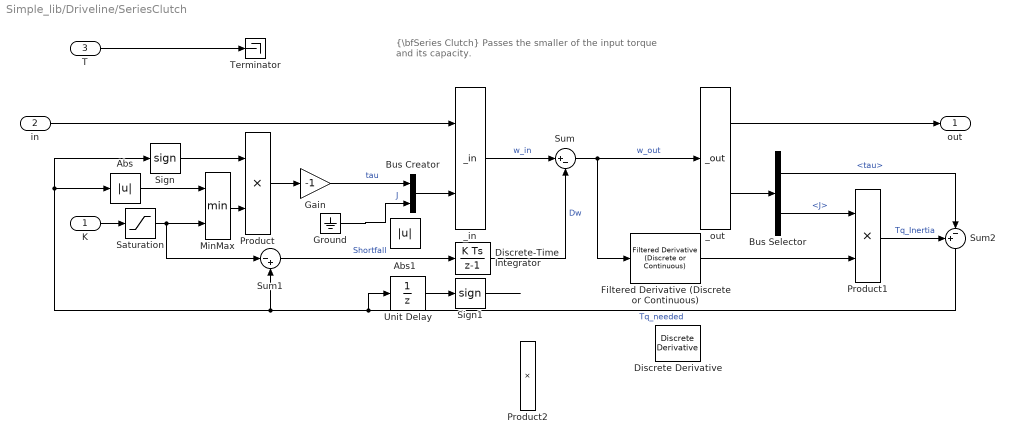
== system Simple_lib/Driveline/SeriesClutch ==
  note: {\bfSeries Clutch}
      | Passes the smaller of the input torque and its capacity.
  K : Inport
  in : Inport  Port=2
  T : Inport  Port=3
  Abs : Abs
  Abs1 : Abs
  Bus Creator : BusCreator  Inputs=2
  Bus Selector : BusSelector  OutputSignals=tau,J
  Discrete Derivative : simulink/Discrete/Discrete Derivative  gainval=1.0  ICPrevScaledInput=0.0  OutMin=[]  OutMax=[]  OutDataType=fixdt(1, 16)  OutScaling=2^-10  DoSatur=off
  Discrete-Time Integrator : DiscreteIntegrator  gainval=20  SampleTime=Ts  LimitOutput=on  LowerSaturationLimit=0  ICPrevOutput=DiscIntNeverNeededParam  ICPrevScaledInput=DiscIntNeverNeededParam
  Filtered Derivative (Discrete or Continuous) : peGeneralControl/Filtered Derivative (Discrete or Continuous)  K=1  T=Ts*100  B=inf  A=-inf  minRatio=10  Ts=-1
  Gain : Gain  Gain=-1
  Ground : Ground
  MinMax : MinMax  Inputs=2
  Product : Product
  Product1 : Product
  Product2 : Product
  Saturation : Saturate  UpperLimit=inf  LowerLimit=0
      settings: AttributesFormatString=|
      | %<UpperLimit>
      | %<LowerLimit>
  Sign : Signum
  Sign1 : Signum
  Sum : Sum  Inputs=|+-
  Sum1 : Sum  Inputs=|-+
  Sum2 : Sum  Inputs=+-|
  Terminator : Terminator
  Unit Delay : UnitDelay  SampleTime=-1
  _in : $bdroot/Rotational/_in  Level=w  Flow=Tq
  _out : $bdroot/Rotational/_out  Tag=Electrical  Level=w  Flow=Tq
  out : Outport
  wires:
  Unit Delay/1 -> Sign1/1
  Sign1/1 -> ?
  Sum/1 -> _out/1, Filtered Derivative (Discrete or Continuous)/1  "w_out"
  _in/1 -> Sum/1  "w_in"
  Gain/1 -> Bus Creator/1  "tau"
  Bus Selector/1 -> Sum2/2  "<tau>"
  Product1/1 -> Sum2/1  "Tq_Inertia"
  Bus Selector/2 -> Product1/1  "<J>"
  Filtered Derivative (Discrete or Continuous)/1 -> Product1/2
  Ground/1 -> Bus Creator/2  "J"
  _out/2 -> Bus Selector/1
  Bus Creator/1 -> _in/2
  _out/1 -> out/1
  MinMax/1 -> Product/2
  K/1 -> Saturation/1
  Abs/1 -> MinMax/1
  Product/1 -> Gain/1
  Sign/1 -> Product/1
  Sum1/1 -> Discrete-Time Integrator/1  "Shortfall"
  Discrete-Time Integrator/1 -> Sum/2  "Dw"
  in/1 -> _in/1
  Saturation/1 -> Sum1/1, MinMax/2
  T/1 -> Terminator/1
  Sum2/1 -> Sum1/2, Abs/1, Sign/1, Unit Delay/1  "Tq_needed"

== system Simple_lib/Driveline/Shaft ==
  In1 : Inport
  SpringDamper : $bdroot/Rotational/SpringDamper  k_spring=1  b_damper=0  b_spring=inf  I_out=0  I_split=0  w_0=w_0  theta_0=0
  Out1 : Outport
  wires:
  SpringDamper/1 -> Out1/1
  In1/1 -> SpringDamper/1

== system Simple_lib/Driveline/Sprag ==
  In1 : Inport
  Bus Selector : BusSelector  OutputSignals=tau
  Discrete-Time Integrator1 : DiscreteIntegrator  gainval=1/0.01  InitialCondition=-deltaV  SampleTime=Ts  LimitOutput=on  LowerSaturationLimit=-deltaV  ICPrevOutput=DiscIntNeverNeededParam  ICPrevScaledInput=DiscIntNeverNeededParam
  Sum : Sum  Inputs=|++
  in : $bdroot/Rotational/_in  Level=w  Flow=Tq
  out : $bdroot/Rotational/_out  Tag=Electrical  Level=w  Flow=Tq
  Out1 : Outport
  wires:
  Discrete-Time Integrator1/1 -> Sum/2
  out/1 -> Out1/1
  Sum/1 -> out/1
  out/2 -> Bus Selector/1, in/2
  in/1 -> Sum/1
  In1/1 -> in/1
  Bus Selector/1 -> Discrete-Time Integrator1/1  "<tau>"

== system Simple_lib/Driveline/SteeredWheel ==
  str : Inport
  brk : Inport  Port=2
  rot : Inport  Port=3
  psn : Inport  Port=4
  Bus Creator : BusCreator  Inputs=4
  Bus Creator1 : BusCreator  Inputs=2
  Ground : $bdroot/Driveline/Grnd  SystemSampleTime=-1
  Hub : $bdroot/Driveline/Hub  I=1
  Suspension : $bdroot/Driveline/Suspension  k=20e3  b=2e3  I=10  v_0=0
  Tyre : $bdroot/Driveline/Tyre  k_lin=2e5  b_lin=1e4  r_0=0.30  I=0.2
  wires:
  rot/1 -> Bus Creator/3  "rtn"
  Tyre/1 -> Ground/1
  Suspension/1 -> Bus Creator/4  "trn"
  psn/1 -> Suspension/1
  str/1 -> Bus Creator/1  "str"
  Hub/1 -> Bus Creator1/1  "hub"
  brk/1 -> Bus Creator/2  "brk"
  Bus Creator/1 -> Hub/1
  Bus Creator1/1 -> Tyre/1
  Ground/1 -> Bus Creator1/2  "gnd"

== system Simple_lib/Driveline/Suspension ==
  In1 : Inport
  Bus Creator : BusCreator  Inputs=3
  Bus Selector : BusSelector  OutputSignals=i,j,k
  SpringDamper : $bdroot/Translational/SpringDamper  k_spring=1000  b_damper=0  b_spring=inf  m_out=0  m_split=0  v_0=v_0  s_0=0
  Out1 : Outport
  wires:
  SpringDamper/1 -> Bus Creator/3  "k"
  Bus Selector/3 -> SpringDamper/1  "<k>"
  Bus Selector/2 -> Bus Creator/2  "<j>"
  Bus Creator/1 -> Out1/1
  In1/1 -> Bus Selector/1
  Bus Selector/1 -> Bus Creator/1  "<i>"

== system Simple_lib/Driveline/Synchro ==
  w_in : Inport
  cap : Inport  Port=2
  w_out : Inport  Port=3
  1/R1 : Gain  Gain=-1
  1/R4 : Gain  Gain=-1
  Delay : Delay  DelayLength=1  InitialCondition=0
  Dynamic Friction : Subsystem
  Push_in : PlantUtilityBlockset_lib/Utility/Push  SystemSampleTime=-1
  Push_out : PlantUtilityBlockset_lib/Utility/Push  SystemSampleTime=-1
  Static Friction : Subsystem
  Sum : Sum  Inputs=+|+
  Sum1 : Sum  Inputs=+|+
  wires:
  1/R1/1 -> Push_out/2
  cap/1 -> Static Friction/1(cap), Dynamic Friction/2(cap)
  Delay/1 -> Static Friction/4(Tq)
  Static Friction/1(Tq_stat) -> Sum1/2
  Dynamic Friction/1(Tq_dyn) -> Sum1/1
  Push_in/1 -> 1/R4/1
  Push_out/1 -> Sum/2, Static Friction/3(w)
  Sum/1 -> Static Friction/2(Dw), Dynamic Friction/1(Dw)
  Sum1/1 -> Push_in/2, Delay/1, 1/R1/1
  1/R4/1 -> Sum/1
  w_in/1 -> Push_in/1
  w_out/1 -> Push_out/1

== system Simple_lib/Driveline/Synchro1 ==
  w_in : Inport
  cap : Inport  Port=2
  w_out : Inport  Port=3
  1/R1 : Gain  Gain=-1
  1/R4 : Gain  Gain=-1
  Delay : Delay  DelayLength=1  InitialCondition=0
  Dw : Scope
  Dynamic Friction : Subsystem
  Push_in : $bdroot/Utility/Input  Level=V  Flow=I
  Push_out : $bdroot/Utility/Input  Level=V  Flow=I
  Static Friction : Subsystem
  Sum : Sum  Inputs=+|+
  Sum1 : Sum  Inputs=+|+
  Tq_Dyn : Scope
  Tq_stat : Scope
  Tq_trans : Scope
  capacity : Scope
  wires:
  w_out/1 -> Push_out/1
  w_in/1 -> Push_in/1
  1/R4/1 -> Sum/1
  Sum1/1 -> 1/R1/1, Delay/1, Push_in/2
  Sum/1 -> Dynamic Friction/1(Dw), Dw/1, Static Friction/2(Dw)
  Push_out/1 -> Static Friction/3(w), Sum/2
  Push_in/1 -> 1/R4/1
  Dynamic Friction/1(Tq_dyn) -> Tq_Dyn/1, Sum1/1
  Static Friction/1(Tq_stat) -> Tq_stat/1, Sum1/2
  Delay/1 -> Tq_trans/1, Static Friction/4(Tq)
  cap/1 -> capacity/1, Dynamic Friction/2(cap), Static Friction/1(cap)
  1/R1/1 -> Push_out/2

== system Simple_lib/Driveline/Synchro2 ==
  note: need (?) spring; mass; friction function 'damper'
  closure : Inport  Tag=NOFLUX
  In1 : Inport  Port=2
  In2 : Inport  Port=3
  1/R1 : Gain  Gain=-1
  1/R4 : Gain  Gain=-1
  Mux : Mux  Inputs=2
  Product : Product  RndMeth=Zero
  Sum : Sum  Inputs=+|+
  capacity : Gain  Gain=100
  fluxIn1Gain : Gain  SaturateOnIntegerOverflow=on  OutDataTypeStr=Inherit: Same as input  ParamDataTypeStr=Inherit: Same as input
  fluxIn2Gain : Gain  SaturateOnIntegerOverflow=on  OutDataTypeStr=Inherit: Same as input  ParamDataTypeStr=Inherit: Same as input
  friction : Trigonometry  Operator=tanh
  grab : Gain  Gain=.01
  tauDisplay : Display
  tauSynchro : Scope
  wsSynchro2 : Scope
  tag scope: fluxIn1Synchro2CanManTran1=global, fluxIn2Synchro2CanManTran1=global
  wires:
  In1/1 -> 1/R4/1, Mux/1
  fluxIn1Gain/1 -> [fluxIn1Synchro2CanManTran1]
  fluxIn2Gain/1 -> [fluxIn2Synchro2CanManTran1]
  In2/1 -> Sum/2, Mux/2
  Sum/1 -> grab/1
  grab/1 -> friction/1
  friction/1 -> Product/1
  Product/1 -> 1/R1/1, fluxIn1Gain/1
  closure/1 -> capacity/1
  1/R1/1 -> fluxIn2Gain/1, tauSynchro/1, tauDisplay/1
  1/R4/1 -> Sum/1
  capacity/1 -> Product/2
  Mux/1 -> wsSynchro2/1

== system Simple_lib/Driveline/Torque Source ==
  w : Inport
  tau : Inport  Port=2
  Simplex : Subsystem  Tag=Driveline  AncestorBlock=PlantUtilityBlockset_lib/Utility/Simplex  InitFcn=initSimplex
      mask Display:
      | color('white')
      | plot([0 3], [2 2])
      | plot([0 3], [-2 -2])
      | color('black')
      | 
      | plot([0 2 2 3], [1 1 0 0])
      | plot([1 3 2 1 0 2], [0.6 0.6 0.4 0.6 0.4 0.4])
      | patch([1 3 2],[0.6 0.6 0.4],[0,0,0])
      | plot([0 1 1], [1 1 0.6])
      | plot([1 1 0], [0.4 -1 -1])
  Terminator : Terminator
  wires:
  Simplex/1(OutPot) -> Terminator/1
  w/1 -> Simplex/1(InPot)
  tau/1 -> Simplex/2(InFlow)

== system Simple_lib/Driveline/Transfer Case ==
  in : Inport
  ctrl : Inport  Port=2
  Clutch : $bdroot/Driveline/Clutch  w_0=0  grab=.1  I=0
  Ground : Ground
  Rear : Outport
  Front : Outport  Port=2
  wires:
  Ground/1 -> Clutch/3
  ctrl/1 -> Clutch/1
  in/1 -> Rear/1, Clutch/2
  Clutch/1 -> Front/1

== system Simple_lib/Driveline/Transmission ==
  In1 : Inport
  Gear1 : $bdroot/Driveline/GearPair  n_i=100  n_o=r*100
  Out1 : Outport
  wires:
  Gear1/1 -> Out1/1
  In1/1 -> Gear1/1

== system Simple_lib/Driveline/Tyre ==
  in : Inport
  BiGain : $bdroot/Translational/BiGain  k_level=-1  k_flow=-1
      settings: AttributesFormatString="%<k_flow>   %<k_level>"
  Bus Creator : BusCreator  Inputs=2
  Bus Selector : BusSelector  OutputSignals=k
  Bus Selector1 : BusSelector  OutputSignals=i,j
  Bus Selector2 : BusSelector  OutputSignals=hub,gnd
  Bus Selector3 : BusSelector  OutputSignals=rtn,trn
  Bus Selector4 : BusSelector  OutputSignals=hub
  Bus Selector5 : BusSelector  OutputSignals=trn
  Compliance : $bdroot/Translational/Stiffness  k_spring=1000  s_0=0  I_spring=0  b_series=inf
  Contact : $bdroot/Driveline/Compliant Wheel_wv  SystemSampleTime=-1
  Damping : $bdroot/Translational/Damping  b=b_lin
  Eqbm Radius : Constant  Value=r_0
  SpringDamper : $bdroot/Translational/SpringDamper  k_spring=1000  b_damper=0  b_spring=inf  m_out=0  m_split=0  v_0=0  s_0=0
  Sum : Sum  Inputs=|+-
  Sum1 : Sum  Inputs=++|
  out : Outport
  wires:
  Bus Selector5/1 -> Bus Selector1/1  "<trn>"
  Bus Selector4/1 -> Bus Selector5/1  "<hub>"
  Bus Selector3/2 -> Bus Selector/1  "<trn>"
  Bus Selector2/1 -> Bus Selector3/1  "<hub>"
  Sum1/1 -> Bus Creator/1  "i"
  Contact/1 -> BiGain/1
  Bus Selector1/2 -> Bus Creator/2  "<j>"
  Bus Selector1/1 -> Sum1/2  "<i>"
  Sum/1 -> Contact/2
  Compliance/1 -> Sum/2
  Bus Selector3/1 -> SpringDamper/1  "<rtn>"
  Eqbm Radius/1 -> Sum/1
  Bus Creator/1 -> out/1  "hrz"
  Bus Selector/1 -> Compliance/2, Damping/2  "<k>"
  in/1 -> Bus Selector2/1, Bus Selector4/1
  Bus Selector2/2 -> Compliance/1, Damping/1  "<gnd>"
  BiGain/1 -> Sum1/1
  SpringDamper/1 -> Contact/1

== system Simple_lib/Driveline/Tyre1 ==
  in : Inport
  Bus Creator : BusCreator  Inputs=2
  Bus Selector1 : BusSelector  OutputSignals=hub.rtn,hub.trn.k,dz,hub.trn.i,hub.trn.j
  Compliance : $bdroot/Mechanics/Stiffness  k=100
  Contact : $bdroot/Driveline/Compliant Wheel_wv  SystemSampleTime=-1
  Damping : $bdroot/Mechanics/Damping  b=2*sqrt(100*.1)
  Eqbm Radius : Constant  Value=0.3
  Sum : Sum  Inputs=|++
  Sum1 : Sum  Inputs=++|
  out : Outport
  wires:
  Sum1/1 -> Bus Creator/1  "i"
  Contact/1 -> Sum1/1
  Bus Selector1/5 -> Bus Creator/2  "<j>"
  Bus Selector1/4 -> Sum1/2  "<i>"
  Sum/1 -> Contact/2
  Compliance/1 -> Sum/2
  Bus Selector1/1 -> Contact/1  "<rtn>"
  Eqbm Radius/1 -> Sum/1
  Bus Creator/1 -> out/1  "hrz"
  Bus Selector1/2 -> Compliance/2, Damping/2  "<k>"
  in/1 -> Bus Selector1/1
  Bus Selector1/3 -> Compliance/1, Damping/1  "<dz>"

== system Simple_lib/Driveline/Wheel ==
  brk : Inport
  rot : Inport  Port=2
  psn : Inport  Port=3
  Bus Creator : BusCreator  Inputs=4
  Bus Creator1 : BusCreator  Inputs=2
  Ground : $bdroot/Driveline/Grnd  SystemSampleTime=-1
  Ground1 : Ground
  Hub : $bdroot/Driveline/Hub  I=1
  Suspension : $bdroot/Driveline/Suspension  k=20000  b=2000  I=10  v_0=0
  Tyre : $bdroot/Driveline/Tyre  k_lin=2e5  b_lin=1e4  r_0=0.30  I=0.4
  wires:
  Ground/1 -> Bus Creator1/2  "gnd"
  Tyre/1 -> Ground/1
  rot/1 -> Bus Creator/3  "rtn"
  Bus Creator1/1 -> Tyre/1
  Hub/1 -> Bus Creator1/1  "hub"
  brk/1 -> Bus Creator/2  "brk"
  Ground1/1 -> Bus Creator/1  "str"
  Suspension/1 -> Bus Creator/4  "trn"
  psn/1 -> Suspension/1
  Bus Creator/1 -> Hub/1

== system Simple_lib/Driveline/Wheel_vw ==
  v : Inport
  1/r : Gain  Gain=1/0.3
  1/radius : Gain  Gain=1/0.3
  Pull : $bdroot/Utility/Output  Tag=Electrical  Level=Level  Flow=flow
  Push : $bdroot/Utility/Input  Level=V  Flow=I
  Sum : Sum  Inputs=+
  w : Outport
  wires:
  Push/1 -> 1/radius/1
  1/radius/1 -> Pull/1
  Pull/2 -> Sum/1
  1/r/1 -> Push/2
  v/1 -> Push/1
  Pull/1 -> w/1
  Sum/1 -> 1/r/1

== system Simple_lib/Driveline/Wheel_wv ==
  w : Inport
  Pull : $bdroot/Utility/Output  Tag=Electrical  Level=Level  Flow=flow
  Push : $bdroot/Utility/Input  Level=V  Flow=I
  Sum : Sum  Inputs=+
  r : Gain  Gain=0.3
  radius : Gain  Gain=0.3
  v : Outport
  wires:
  Push/1 -> radius/1
  radius/1 -> Pull/1
  Pull/2 -> Sum/1
  r/1 -> Push/2
  w/1 -> Push/1
  Pull/1 -> v/1
  Sum/1 -> r/1

== system Simple_lib/Driveline/diff_R ==
  w_in_1 : Inport
  w_in_2 : Inport  Port=2
  Carrier : Subsystem  InitFcn=bond  mask{n_i=37, n_o=23}
      mask prompts: n_i "Number of input teeth"; n_o "Number of output teeth"
      mask Display:
      | color('white')
      | plot([-1 1], [1 1]);
      | plot([-1 1], [-1 -1]);
      | 
      | color('black')
      | plot([-1 1], [0.5 0.5]);
      | plot([1 1], [0.5 0.2]);
      | plot([-1 1],[0 0]);
      | plot([1 1], [-0.5 -0.2]);
      | plot([-1 1],[-.5 -.5]);
      | 
      | %port_label('input', 1, 'a')
      | %port_label('input', 2, 's')
  "GearPair " : Subsystem  AncestorBlock=PlantUtilityBlockset_lib/Driveline/GearPair  mask{n_i=37, n_o=23}
      mask prompts: n_i "Number of input teeth"; n_o "Number of output teeth"
      mask Display:
      | plot([-n_i -1],[0 0]);
      | plot([1 n_o],[0 0]);
      | plot([-1 -1],[-(n_i+n_o)  (n_i+n_o)]);
      | plot([1 1],[-(n_i+n_o)  (n_i+n_o)]);
      | %plot([n_o n_o+6 n_o+6 n_o],[0 10 -10 0  ])
  GearPair 1 : Subsystem  AncestorBlock=PlantUtilityBlockset_lib/Driveline/GearPair  mask{n_i=37, n_o=23}
      mask prompts: n_i "Number of input teeth"; n_o "Number of output teeth"
      mask Display:
      | plot([-n_i -1],[0 0]);
      | plot([1 n_o],[0 0]);
      | plot([-1 -1],[-(n_i+n_o)  (n_i+n_o)]);
      | plot([1 1],[-(n_i+n_o)  (n_i+n_o)]);
      | %plot([n_o n_o+6 n_o+6 n_o],[0 10 -10 0  ])
  w_out : Outport
  wires:
  Carrier/1(w_out) -> w_out/1
  w_in_1/1 -> "GearPair "/1(In1)
  w_in_2/1 -> GearPair 1/1(In1)
  "GearPair "/1(Out1) -> Carrier/1(w_in_1)
  GearPair 1/1(Out1) -> Carrier/2(w_in_2)

== system Simple_lib/Driveline/lev ==
  v : Inport
  Bus Creator : BusCreator  Inputs=2
  Bus Selector : BusSelector  OutputSignals=tau,J
  Gain{,1..3} (4 alike) : Gain  Gain=1/r
  _in : $bdroot/Translational/_in  Level=v  Flow=F
  _out : $bdroot/Rotational/_out  Tag=Electrical  Level=w  Flow=tau
  w : Outport
  wires:
  Gain2/1 -> Gain3/1
  Gain3/1 -> Bus Creator/2  "M"
  Gain1/1 -> Bus Creator/1  "F"
  _out/1 -> w/1
  v/1 -> _in/1
  Bus Creator/1 -> _in/2
  _out/2 -> Bus Selector/1
  Gain/1 -> _out/1
  _in/1 -> Gain/1
  Bus Selector/2 -> Gain2/1  "<J>"
  Bus Selector/1 -> Gain1/1  "<tau>"

== system Simple_lib/Driveline/rev ==
  w : Inport
  Bus Creator : BusCreator  Inputs=2
  Bus Selector : BusSelector  OutputSignals=F,M
  Gain{,1..3} (4 alike) : Gain  Gain=r
  _in : $bdroot/Rotational/_in  Level=w  Flow=tau
  _out : $bdroot/Translational/_out  Tag=Electrical  Level=v  Flow=F
  v : Outport
  wires:
  Bus Selector/1 -> Gain1/1  "<F>"
  Bus Selector/2 -> Gain2/1  "<M>"
  _in/1 -> Gain/1
  Gain/1 -> _out/1
  _out/2 -> Bus Selector/1
  Bus Creator/1 -> _in/2
  w/1 -> _in/1
  _out/1 -> v/1
  Gain1/1 -> Bus Creator/1  "tau"
  Gain3/1 -> Bus Creator/2  "J"
  Gain2/1 -> Gain3/1

== system Simple_lib/Electrical/B ==
  In1 : Inport
  C0 : PlantUtilityBlockset_lib/Electrical/C0  C=0.1
  E1 : PlantUtilityBlockset_lib/Electrical/E  SystemSampleTime=-1
  L1 : PlantUtilityBlockset_lib/Electrical/L1  L=1
  R1 : PlantUtilityBlockset_lib/Electrical/R  R=1
  Out1 : Outport
  wires:
  C0/1 -> L1/1, R1/1
  In1/1 -> E1/1
  R1/1 -> Out1/1
  E1/1 -> L1/2

== system Simple_lib/Electrical/B0 ==
  In1 : Inport
  In2 : Inport  Port=2
  E1 : PlantUtilityBlockset_lib/Electrical/E  SystemSampleTime=-1
  L1 : PlantUtilityBlockset_lib/Electrical/L1  L=1
  R1 : PlantUtilityBlockset_lib/Electrical/R  R=0.01
  wires:
  In1/1 -> E1/1
  E1/1 -> L1/2
  R1/1 -> L1/1
  In2/1 -> R1/1

== system Simple_lib/Electrical/B2 ==
  In1 : Inport
  C : Subsystem
      mask Display:
      | %% something
      | %color('red');
      | %patch([0 10 20 30 30 0], [10 30 20 25 10 10],[1 1 1])
      | %port_label('output',1,get(gcbh,'Name'))
      | 
      | plot([0 1], [0.3 0.3])
      | plot([0 1], [0.5 0.5])
      | plot([0.2 0.8], [0.2 0.2])
      | plot([0.4 0.6], [0.1 0.1])
      | 
      | plot([0.5 0.5], [0 0.3])
      | plot([0.5 0.5], [0.5 1])
  E : Subsystem
      mask Display:
      | plot([-1 -1], [-0.5 0.5])
      | plot([1 1], [-1 1.0])
  L : Subsystem
      mask Display:
      | color('white')
      | plot([-1 -1], [-1 1])
      | color('black')
      | 
      | plot(   [    0     0.3827     0.7071     0.9239     1.0000     0.9239     0.7071     0.3827     0.0000    -0.3827    -0.7071    -0.9239    -1.0000    -0.9239    -0.7071    -0.3827    -0.0000     0.3827     0.7071     0.9239     1.0000     0.9239     0.7071     0.3827     0.0000    -0.3827    -0.7071    -0.9239    -1.0000    -0.9239    -0.7071    -0.3827    -0.0000     0.3827     0.7071     0.9239     1.0000     0.9239     0.7071     0.3827     0.0000    -0.3827    -0.7071    -0.9239    -1.0000    -0.9239    -0.7071    -0.3827    -0.0000     0.3827     0.7071     0.9239     1.0000     0.9239     0.7071     0.3827     0.0000    -0.3827    -0.7071    -0.9239    -1.0000    -0.9239    -0.7071    -0.3827    -0.0000],   -.5+[-0.0625    -0.0421    -0.0129     0.0230     0.0625     0.1020     0.1379     0.1671     0.1875     0.1984     0.2004     0.1958     0.1875     0.1792     0.1746     0.1766     0.1875     0.2079     0.2371     0.2730     0.3125     0.3520     0.3879     0.4171     0.4375     0.4484     0.4504     0.4458     0.4375     0.4292     0.4246     0.4266     0.4375     0.4579     0.4871     0.5230     0.5625     0.6020     0.6379     0.6671     0.6875     0.6984     0.7004     0.6958     0.6875     0.6792     0.6746     0.6766     0.6875     0.7079     0.7371     0.7730     0.8125     0.8520     0.8879     0.9171     0.9375     0.9484     0.9504     0.9458     0.9375     0.9292     0.9246     0.9266     0.9375])
  R0 : Subsystem  AncestorBlock=Electrical_lib/R  mask{R=.01}
      mask prompts: R "Resistance (Ohms)"
      mask Display: plot([0:16]/16, [0 1 0 -1 0 1 0 -1 0 1 0 -1 0 1 0 -1 0]/2+.5)
  Out1 : Outport
  wires:
  C/1(J1) -> L/2(In2), R0/1(In1)
  In1/1 -> E/1(In1)
  R0/1(Out1) -> Out1/1
  E/1(Out1) -> L/1(In1)
